simulink model "Operational_SpacePD"  (R2016a)
settings: Solver=VariableStepAuto  StartTime=0.0  StopTime=t_d  RelTol=1e-3
values from neighbouring files (symbols this model uses):
  F_v = K_r*diag([0.01 0.01])*K_r    [i8_15.m]
  g = 9.81    [i8_15.m]
  K_d = 750*diag([1 1])    [i8_15.m]
  K_p = 3750*diag([1 1])    [i8_15.m]
  pi_l = pi_m    [i8_15.m]
  Tc = 0.001    [i8_15.m]
  Ts = Tc    (= 0.001)    [i8_15.m]
  x_d = [0.6; -0.2]    [i8_15.m]
undefined symbols (not defined in the file or in its folder): a, iner_l, pi_m
settings Model: Creator=Prabal  LastModifiedBy=Prabal

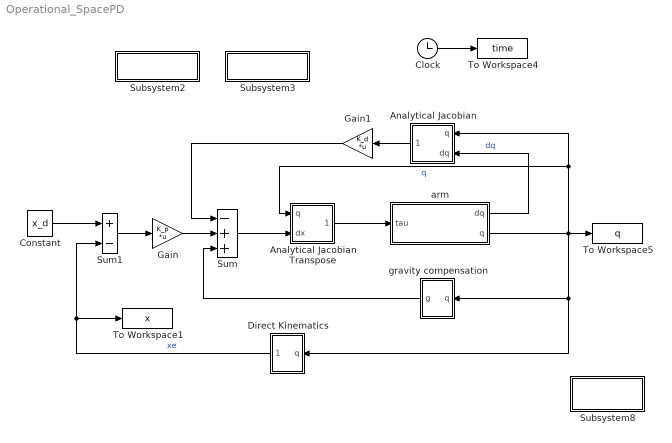
== system Operational_SpacePD ==
  Analytical Jacobian : Subsystem
      mask Display: disp('JA(q)')
  Analytical Jacobian Transpose : Subsystem
      mask Display: disp('JA"(q)')
  Clock : Clock
  Constant : Constant  Value=x_d
  Direct Kinematics : Subsystem
      mask Display: disp('k(q)')
  Gain : Gain  Gain=K_p  Multiplication=Matrix(K*u)  SampleTime=Tc
      mask Display: disp('K_p')
  Gain1 : Gain  Gain=K_d  Multiplication=Matrix(K*u)  SampleTime=Tc
      mask Display: disp('K_d')
  Subsystem2 : Subsystem
      settings: OpenFcn=clear all;c=0;i8_10;
      mask Display: disp('x_d=[0.5 0.5]')
  Subsystem3 : Subsystem
      settings: OpenFcn=clear all;c=1;i8_10;
      mask Display: disp('x_d=[0.6 -0.2]')
  Subsystem8 : Subsystem
      settings: OpenFcn=p8_15;
      mask Display: disp('plot')
  Sum : Sum  Inputs=-++  SaturateOnIntegerOverflow=on  InputSameDT=on  OutDataTypeStr=Inherit: Same as first input
  Sum1 : Sum  Inputs=+-  SampleTime=Tc  SaturateOnIntegerOverflow=on  InputSameDT=on  OutDataTypeStr=Inherit: Same as first input
  To Workspace1 : ToWorkspace  VariableName=x  SampleTime=Ts
      settings: MaxDataPoints=4001
  To Workspace4 : ToWorkspace  VariableName=time  SampleTime=Ts
      settings: MaxDataPoints=4001
  To Workspace5 : ToWorkspace  VariableName=q  SampleTime=Ts
      settings: MaxDataPoints=4001
  arm : Subsystem
      mask Display: disp('inv(B(q))(tau-tau'')')
  gravity compensation : Subsystem
      mask Display: disp('g(q)')
  wires:
  Sum/1 -> Analytical Jacobian Transpose/2(dx)
  Gain1/1 -> Sum/1
  Sum1/1 -> Gain/1
  Clock/1 -> To Workspace4/1
  Gain/1 -> Sum/2
  gravity compensation/1(g) -> Sum/3
  Constant/1 -> Sum1/1
  arm/2("q ") -> gravity compensation/1(q), Direct Kinematics/1(q), To Workspace5/1, Analytical Jacobian Transpose/1(q), Analytical Jacobian/1(q)  "q"
  Direct Kinematics/1(xe) -> Sum1/2, To Workspace1/1  "xe"
  Analytical Jacobian/1(xpdot) -> Gain1/1
  arm/1(dq) -> Analytical Jacobian/2(dq)  "dq"
  Analytical Jacobian Transpose/1(xpdot) -> arm/1(tau)

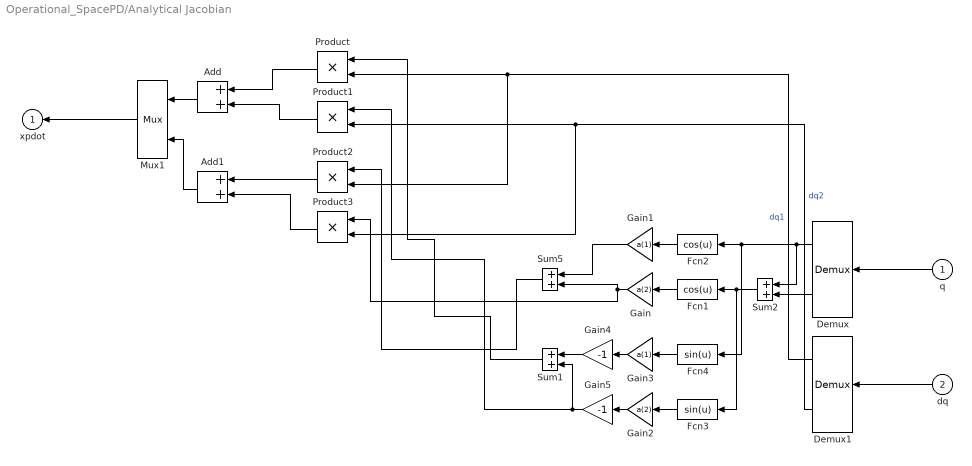
== system Operational_SpacePD/Analytical Jacobian ==
  q : Inport
  dq : Inport  Port=2
  Add : Sum
  Add1 : Sum
  Demux : Demux  Outputs=2
  Demux1 : Demux  Outputs=2
  Fcn1 : Fcn  Expr=cos(u)  SampleTime=Tc
  Fcn2 : Fcn  Expr=cos(u)  SampleTime=Tc
  Fcn3 : Fcn  Expr=sin(u)  SampleTime=Tc
  Fcn4 : Fcn  Expr=sin(u)  SampleTime=Tc
  Gain : Gain  Gain=a(2)  SaturateOnIntegerOverflow=on  OutDataTypeStr=Inherit: Same as input  ParamDataTypeStr=Inherit: Same as input
      mask Display: disp('a_2')
  Gain1 : Gain  Gain=a(1)  SaturateOnIntegerOverflow=on  OutDataTypeStr=Inherit: Same as input  ParamDataTypeStr=Inherit: Same as input
      mask Display: disp('a_1')
  Gain2 : Gain  Gain=a(2)  SaturateOnIntegerOverflow=on  OutDataTypeStr=Inherit: Same as input  ParamDataTypeStr=Inherit: Same as input
      mask Display: disp('a_2')
  Gain3 : Gain  Gain=a(1)  SaturateOnIntegerOverflow=on  OutDataTypeStr=Inherit: Same as input  ParamDataTypeStr=Inherit: Same as input
      mask Display: disp('a_1')
  Gain4 : Gain  Gain=-1
  Gain5 : Gain  Gain=-1
  Mux1 : Mux  Inputs=2
  Product{,1..3} (4 alike) : Product
  Sum1 : Sum  SaturateOnIntegerOverflow=on  InputSameDT=on  OutDataTypeStr=Inherit: Same as first input
  Sum2 : Sum  SampleTime=Tc  SaturateOnIntegerOverflow=on  InputSameDT=on  OutDataTypeStr=Inherit: Same as first input
  Sum5 : Sum  SaturateOnIntegerOverflow=on  InputSameDT=on  OutDataTypeStr=Inherit: Same as first input
  xpdot : Outport  InitialOutput=0
  wires:
  q/1 -> Demux/1
  Demux/2 -> Sum2/2
  Sum2/1 -> Fcn3/1, Fcn1/1
  Fcn1/1 -> Gain/1
  Fcn2/1 -> Gain1/1
  Demux/1 -> Sum2/1, Fcn4/1, Fcn2/1
  Gain1/1 -> Sum5/1
  Gain/1 -> Product3/1, Sum5/2
  Fcn3/1 -> Gain2/1
  Fcn4/1 -> Gain3/1
  Gain3/1 -> Gain4/1
  Gain2/1 -> Gain5/1
  Gain4/1 -> Sum1/1
  Gain5/1 -> Product1/1, Sum1/2
  Sum1/1 -> Product/1
  Sum5/1 -> Product2/1
  dq/1 -> Demux1/1
  Demux1/1 -> Product2/2, Product/2  "dq1"
  Demux1/2 -> Product3/2, Product1/2  "dq2"
  Product/1 -> Add/1
  Product1/1 -> Add/2
  Add/1 -> Mux1/1
  Product2/1 -> Add1/1
  Product3/1 -> Add1/2
  Add1/1 -> Mux1/2
  Mux1/1 -> xpdot/1

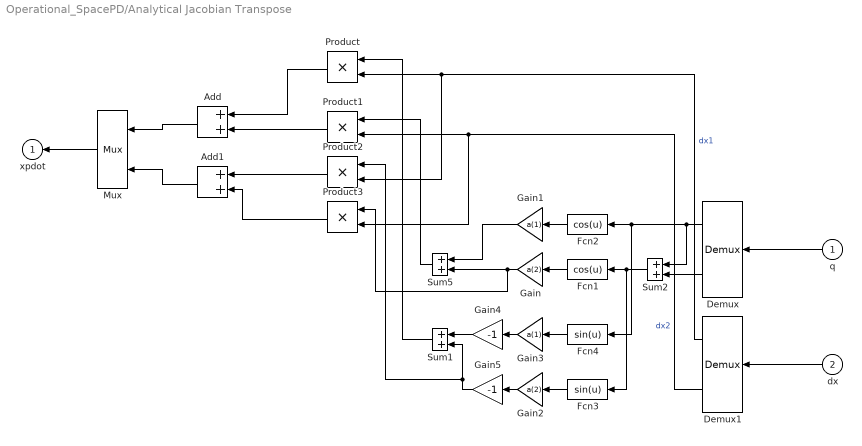
== system Operational_SpacePD/Analytical Jacobian Transpose ==
  q : Inport
  dx : Inport  Port=2
  Add : Sum
  Add1 : Sum
  Demux : Demux  Outputs=2
  Demux1 : Demux  Outputs=2
  Fcn1 : Fcn  Expr=cos(u)  SampleTime=Tc
  Fcn2 : Fcn  Expr=cos(u)  SampleTime=Tc
  Fcn3 : Fcn  Expr=sin(u)  SampleTime=Tc
  Fcn4 : Fcn  Expr=sin(u)  SampleTime=Tc
  Gain : Gain  Gain=a(2)  SaturateOnIntegerOverflow=on  OutDataTypeStr=Inherit: Same as input  ParamDataTypeStr=Inherit: Same as input
      mask Display: disp('a_2')
  Gain1 : Gain  Gain=a(1)  SaturateOnIntegerOverflow=on  OutDataTypeStr=Inherit: Same as input  ParamDataTypeStr=Inherit: Same as input
      mask Display: disp('a_1')
  Gain2 : Gain  Gain=a(2)  SaturateOnIntegerOverflow=on  OutDataTypeStr=Inherit: Same as input  ParamDataTypeStr=Inherit: Same as input
      mask Display: disp('a_2')
  Gain3 : Gain  Gain=a(1)  SaturateOnIntegerOverflow=on  OutDataTypeStr=Inherit: Same as input  ParamDataTypeStr=Inherit: Same as input
      mask Display: disp('a_1')
  Gain4 : Gain  Gain=-1
  Gain5 : Gain  Gain=-1
  Mux : Mux  Inputs=2
  Product{,1..3} (4 alike) : Product
  Sum1 : Sum  SaturateOnIntegerOverflow=on  InputSameDT=on  OutDataTypeStr=Inherit: Same as first input
  Sum2 : Sum  SampleTime=Tc  SaturateOnIntegerOverflow=on  InputSameDT=on  OutDataTypeStr=Inherit: Same as first input
  Sum5 : Sum  SaturateOnIntegerOverflow=on  InputSameDT=on  OutDataTypeStr=Inherit: Same as first input
  xpdot : Outport  InitialOutput=0
  wires:
  Mux/1 -> xpdot/1
  Sum1/1 -> Product/1
  Gain5/1 -> Product2/1, Sum1/2
  Gain4/1 -> Sum1/1
  Gain2/1 -> Gain5/1
  Gain3/1 -> Gain4/1
  Fcn4/1 -> Gain3/1
  Fcn3/1 -> Gain2/1
  Gain/1 -> Sum5/2, Product3/1
  Gain1/1 -> Sum5/1
  Demux/1 -> Fcn2/1, Fcn4/1, Sum2/1
  Fcn2/1 -> Gain1/1
  Fcn1/1 -> Gain/1
  Sum2/1 -> Fcn1/1, Fcn3/1
  Demux/2 -> Sum2/2
  q/1 -> Demux/1
  dx/1 -> Demux1/1
  Product/1 -> Add/1
  Product1/1 -> Add/2
  Add/1 -> Mux/1
  Product2/1 -> Add1/1
  Product3/1 -> Add1/2
  Add1/1 -> Mux/2
  Demux1/1 -> Product2/2, Product/2  "dx1"
  Sum5/1 -> Product1/1
  Demux1/2 -> Product3/2, Product1/2  "dx2"

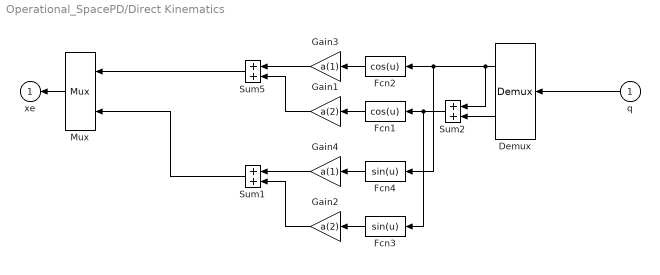
== system Operational_SpacePD/Direct Kinematics ==
  q : Inport
  Demux : Demux  Outputs=2
  Fcn1 : Fcn  Expr=cos(u)  SampleTime=Tc
  Fcn2 : Fcn  Expr=cos(u)  SampleTime=Tc
  Fcn3 : Fcn  Expr=sin(u)  SampleTime=Tc
  Fcn4 : Fcn  Expr=sin(u)  SampleTime=Tc
  Gain1 : Gain  Gain=a(2)
  Gain2 : Gain  Gain=a(2)
  Gain3 : Gain  Gain=a(1)
  Gain4 : Gain  Gain=a(1)
  Mux : Mux  Inputs=2
  Sum1 : Sum  SaturateOnIntegerOverflow=on  InputSameDT=on  OutDataTypeStr=Inherit: Same as first input
  Sum2 : Sum  SampleTime=Tc  SaturateOnIntegerOverflow=on  InputSameDT=on  OutDataTypeStr=Inherit: Same as first input
  Sum5 : Sum  SaturateOnIntegerOverflow=on  InputSameDT=on  OutDataTypeStr=Inherit: Same as first input
  xe : Outport  InitialOutput=0
  wires:
  q/1 -> Demux/1
  Demux/2 -> Sum2/2
  Sum2/1 -> Fcn3/1, Fcn1/1
  Fcn1/1 -> Gain1/1
  Fcn2/1 -> Gain3/1
  Demux/1 -> Fcn4/1, Fcn2/1, Sum2/1
  Gain3/1 -> Sum5/1
  Gain1/1 -> Sum5/2
  Mux/1 -> xe/1
  Sum5/1 -> Mux/1
  Fcn4/1 -> Gain4/1
  Fcn3/1 -> Gain2/1
  Gain4/1 -> Sum1/1
  Gain2/1 -> Sum1/2
  Sum1/1 -> Mux/2

== system Operational_SpacePD/Subsystem2 ==
  note: start

== system Operational_SpacePD/Subsystem3 ==
  note: start

== system Operational_SpacePD/Subsystem8 ==
  note: start

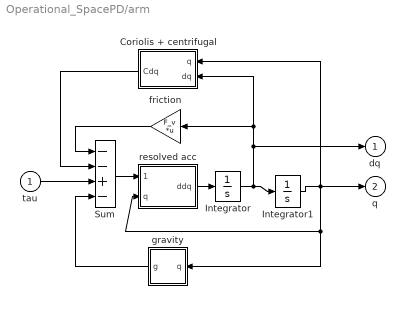
== system Operational_SpacePD/arm ==
  tau : Inport
  Coriolis + centrifugal : Subsystem
      mask Display: disp('C(q,dq)dq')
  Integrator : Integrator  InitialCondition=[0 0]  ZeroCross=off
  Integrator1 : Integrator  InitialCondition=[0.1 0.1]  ZeroCross=off
  Sum : Sum  Inputs=--+-  SaturateOnIntegerOverflow=on  InputSameDT=on  OutDataTypeStr=Inherit: Same as first input
  friction : Gain  Gain=F_v  Multiplication=Matrix(K*u)  SaturateOnIntegerOverflow=on  OutDataTypeStr=Inherit: Same as input  ParamDataTypeStr=Inherit: Same as input
      mask Display: disp('F_v')
  gravity : Subsystem
      mask Display: disp('g(q)')
  resolved acc : Subsystem
      mask Display: disp('inv(B(q))')
  dq : Outport  InitialOutput=0
  "q " : Outport  Port=2  InitialOutput=0
  wires:
  Coriolis + centrifugal/1(Cdq) -> Sum/2
  tau/1 -> Sum/3
  Integrator1/1 -> Coriolis + centrifugal/1(q), resolved acc/2(q), gravity/1(q), "q "/1
  resolved acc/1(ddq) -> Integrator/1
  Integrator/1 -> Integrator1/1, dq/1, Coriolis + centrifugal/2(dq), friction/1
  Sum/1 -> resolved acc/1(tau-tau')
  friction/1 -> Sum/1
  gravity/1(g) -> Sum/4

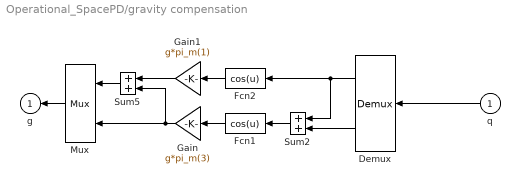
== system Operational_SpacePD/gravity compensation ==
  q : Inport
  Demux : Demux  Outputs=2
  Fcn1 : Fcn  Expr=cos(u)  SampleTime=Tc
  Fcn2 : Fcn  Expr=cos(u)  SampleTime=Tc
  Gain : Gain  Gain=g*pi_m(3)  SaturateOnIntegerOverflow=on  OutDataTypeStr=Inherit: Same as input  ParamDataTypeStr=Inherit: Same as input
      mask Display: disp('k_2')
  Gain1 : Gain  Gain=g*pi_m(1)  SaturateOnIntegerOverflow=on  OutDataTypeStr=Inherit: Same as input  ParamDataTypeStr=Inherit: Same as input
      mask Display: disp('k_1')
  Mux : Mux  Inputs=2
  Sum2 : Sum  SampleTime=Tc  SaturateOnIntegerOverflow=on  InputSameDT=on  OutDataTypeStr=Inherit: Same as first input
  Sum5 : Sum  SaturateOnIntegerOverflow=on  InputSameDT=on  OutDataTypeStr=Inherit: Same as first input
  g : Outport  InitialOutput=0
  wires:
  Mux/1 -> g/1
  Gain/1 -> Sum5/2, Mux/2
  Sum5/1 -> Mux/1
  Gain1/1 -> Sum5/1
  Demux/1 -> Fcn2/1, Sum2/1
  Fcn2/1 -> Gain1/1
  Fcn1/1 -> Gain/1
  Sum2/1 -> Fcn1/1
  Demux/2 -> Sum2/2
  q/1 -> Demux/1

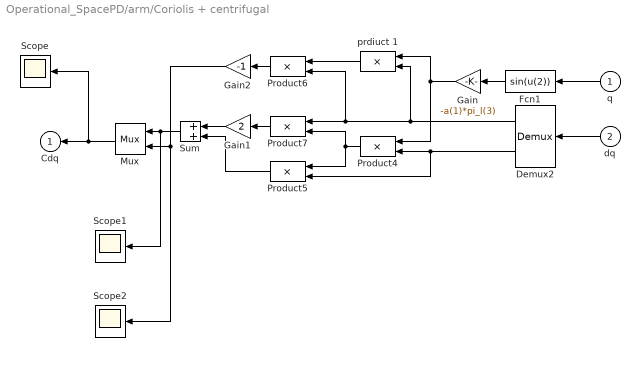
== system Operational_SpacePD/arm/Coriolis + centrifugal ==
  q : Inport
  dq : Inport  Port=2
  Demux2 : Demux  Outputs=2
  Fcn1 : Fcn  Expr=sin(u(2))
  Gain : Gain  Gain=-a(1)*pi_l(3)  SaturateOnIntegerOverflow=on  OutDataTypeStr=Inherit: Same as input  ParamDataTypeStr=Inherit: Same as input
      mask Display: disp('k_3')
  Gain1 : Gain  Gain=2  SaturateOnIntegerOverflow=on  OutDataTypeStr=Inherit: Same as input  ParamDataTypeStr=Inherit: Same as input
  Gain2 : Gain  Gain=-1  SaturateOnIntegerOverflow=on  OutDataTypeStr=Inherit: Same as input  ParamDataTypeStr=Inherit: Same as input
  Mux : Mux  Inputs=2
  Product{4..7} (4 alike) : Product  SaturateOnIntegerOverflow=on  RndMeth=Zero  InputSameDT=on  OutDataTypeStr=Inherit: Same as first input
  Scope : Scope
  Scope1 : Scope
  Scope2 : Scope
  Sum : Sum  SaturateOnIntegerOverflow=on  InputSameDT=on  OutDataTypeStr=Inherit: Same as first input
  prdiuct 1 : Product  SaturateOnIntegerOverflow=on  RndMeth=Zero  InputSameDT=on  OutDataTypeStr=Inherit: Same as first input
  Cdq : Outport  InitialOutput=0
  wires:
  dq/1 -> Demux2/1
  Gain2/1 -> Scope2/1, Mux/2
  Product6/1 -> Gain2/1
  Mux/1 -> Scope/1, Cdq/1
  Sum/1 -> Scope1/1, Mux/1
  Product5/1 -> Sum/2
  Gain1/1 -> Sum/1
  Product7/1 -> Gain1/1
  Demux2/1 -> prdiuct 1/2, Product6/2, Product7/1
  Demux2/2 -> Product4/2, Product5/2
  prdiuct 1/1 -> Product6/1
  Gain/1 -> prdiuct 1/1, Product4/1
  Fcn1/1 -> Gain/1
  q/1 -> Fcn1/1
  Product4/1 -> Product5/1, Product7/2

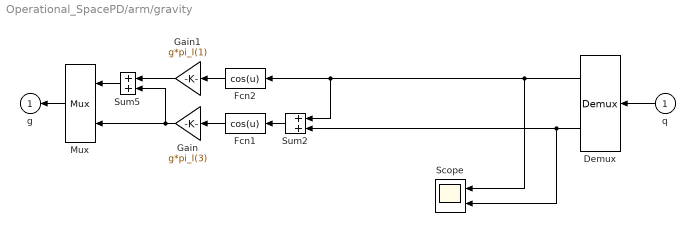
== system Operational_SpacePD/arm/gravity ==
  q : Inport
  Demux : Demux  Outputs=2
  Fcn1 : Fcn  Expr=cos(u)
  Fcn2 : Fcn  Expr=cos(u)
  Gain : Gain  Gain=g*pi_l(3)  SaturateOnIntegerOverflow=on  OutDataTypeStr=Inherit: Same as input  ParamDataTypeStr=Inherit: Same as input
      mask Display: disp('k_2')
  Gain1 : Gain  Gain=g*pi_l(1)  SaturateOnIntegerOverflow=on  OutDataTypeStr=Inherit: Same as input  ParamDataTypeStr=Inherit: Same as input
      mask Display: disp('k_1')
  Mux : Mux  Inputs=2
  Scope : Scope  NumInputPorts=2
  Sum2 : Sum  SaturateOnIntegerOverflow=on  InputSameDT=on  OutDataTypeStr=Inherit: Same as first input
  Sum5 : Sum  SaturateOnIntegerOverflow=on  InputSameDT=on  OutDataTypeStr=Inherit: Same as first input
  g : Outport  InitialOutput=0
  wires:
  q/1 -> Demux/1
  Demux/2 -> Scope/2, Sum2/2
  Sum2/1 -> Fcn1/1
  Fcn1/1 -> Gain/1
  Fcn2/1 -> Gain1/1
  Demux/1 -> Scope/1, Fcn2/1, Sum2/1
  Gain1/1 -> Sum5/1
  Sum5/1 -> Mux/1
  Gain/1 -> Sum5/2, Mux/2
  Mux/1 -> g/1

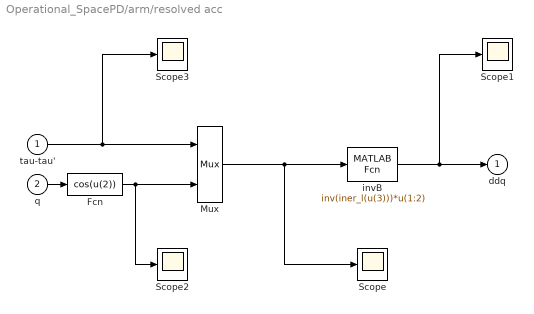
== system Operational_SpacePD/arm/resolved acc ==
  tau-tau' : Inport
  q : Inport  Port=2
  Fcn : Fcn  Expr=cos(u(2))
  Mux : Mux  Inputs=[2,1]
  Scope{,1..3} (4 alike) : Scope
  "invB " : MATLABFcn  MATLABFcn=inv(iner_l(u(3)))*u(1:2)  OutputDimensions=2
      mask Display: disp('inv(B(q))')
  ddq : Outport  InitialOutput=0
  wires:
  Fcn/1 -> Scope2/1, Mux/2
  q/1 -> Fcn/1
  "invB "/1 -> Scope1/1, ddq/1
  tau-tau'/1 -> Scope3/1, Mux/1
  Mux/1 -> Scope/1, "invB "/1
